simulink model "ORC_test_simu"  (R2018a)
settings: Solver=VariableStepAuto  StartTime=0.0  StopTime=10  RelTol=1e-3
undefined symbols (not defined in the file or in its folder): handle_sink, handle_source, handle_wf, sigbuilder_block
libraries: simulink x1
(part 1 of 3)
settings Model: Creator=njgreen3  LastModifiedBy=njgreen3
settings DebuggingCC: ParameterOverflowMsg=warning

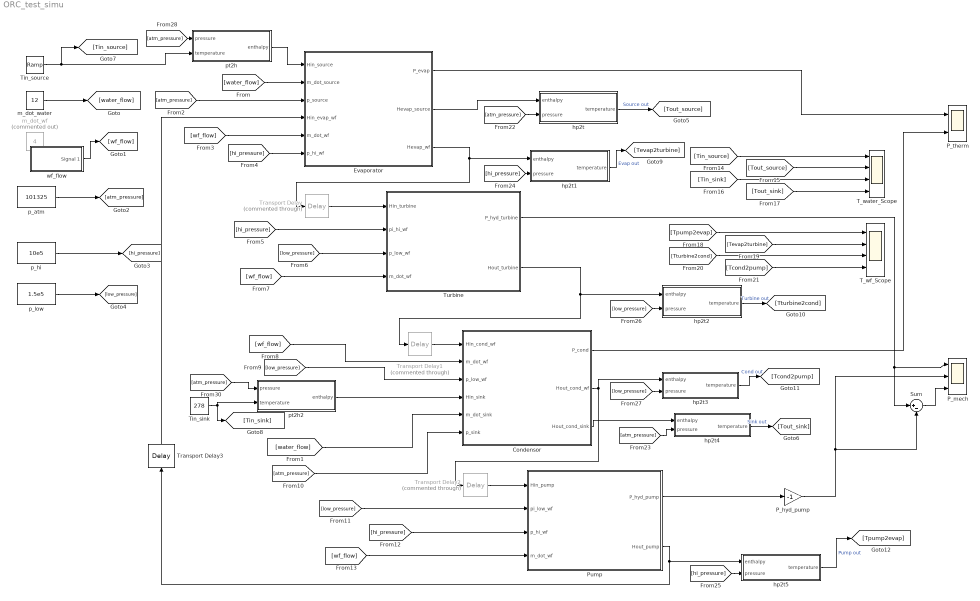
== system ORC_test_simu ==
  Condensor : Subsystem
  Evaporator : Subsystem
  P_hyd_pump : Gain  Gain=-1
  P_mech : Scope  NumInputPorts=3
  P_therm : Scope  NumInputPorts=2
  Pump : Subsystem
  Sum : Sum  Inputs=|+-
  T_water_Scope : Scope  NumInputPorts=4
  T_wf_Scope : Scope  NumInputPorts=4
  Tin_sink : Constant  Value=278
  Tin_source : simulink/Sources/Ramp  slope=0  start=.1  InitialOutput=368
  Transport Delay : TransportDelay  Commented=through  DelayTime=.02  InitialOutput=363
  Transport Delay1 : TransportDelay  Commented=through  DelayTime=.02  InitialOutput=363
  Transport Delay2 : TransportDelay  Commented=through  DelayTime=.02  InitialOutput=306
  Transport Delay3 : TransportDelay  DelayTime=.02  InitialOutput=2.3e+05  TransDelayFeedthrough=on
  Turbine : Subsystem
  hp2t : MATLAB Function  TreatAsAtomicUnit=on  mask{fluid_handle=handle_source}
      mask prompts: fluid_handle "Fluid Handle"
  hp2t1 : MATLAB Function  TreatAsAtomicUnit=on  mask{fluid_handle=handle_wf}
      mask prompts: fluid_handle "Fluid Handle"
  hp2t2 : MATLAB Function  TreatAsAtomicUnit=on  mask{fluid_handle=handle_wf}
      mask prompts: fluid_handle "Fluid Handle"
  hp2t3 : MATLAB Function  TreatAsAtomicUnit=on  mask{fluid_handle=handle_wf}
      mask prompts: fluid_handle "Fluid Handle"
  hp2t4 : MATLAB Function  TreatAsAtomicUnit=on  mask{fluid_handle=handle_sink}
      mask prompts: fluid_handle "Fluid Handle"
  hp2t5 : MATLAB Function  TreatAsAtomicUnit=on  mask{fluid_handle=handle_wf}
      mask prompts: fluid_handle "Fluid Handle"
  m_dot_water : Constant  Value=12
  m_dot_wf : Constant  Commented=on  Value=4
  p_atm : Constant  Value=101325
  p_hi : Constant  Value=10e5
  p_low : Constant  Value=1.5e5
  pt2h : MATLAB Function  TreatAsAtomicUnit=on  mask{fluid_handle=handle_source}
      mask prompts: fluid_handle "Fluid Handle"
  pt2h2 : MATLAB Function  TreatAsAtomicUnit=on  mask{fluid_handle=handle_sink}
      mask prompts: fluid_handle "Fluid Handle"
  wf_flow : Subsystem  Tag=STV Subsys  LoadFcn=sigbuilder_block('load',[319.5 207 550.5 399.75 ]);  StartFcn=sigbuilder_block('start');  StopFcn=sigbuilder_block('stop');  ClipboardFcn=sigbuilder_block('clipboard');  mask(Sigbuilder block){tuvar=[0:10]}
      mask help: Simulink:masks:SigbuilderBlock_MD
      mask init:
      | if ~strcmp(get_param(bdroot(gcbh),'SimulationStatus'),'stopped') tuvar = sigbuilder_block('maskInit'); end
      settings: CopyFcn=sigbuilder_block('copy');  DeleteFcn=sigbuilder_block('delete');  ModelCloseFcn=sigbuilder_block('modelClose');  PreSaveFcn=sigbuilder_block('preSave');  PauseFcn=sigbuilder_block('pause');  ContinueFcn=sigbuilder_block('continue');  NameChangeFcn=sigbuilder_block('namechange');  OpenFcn=sigbuilder_block('open',[437.6 199.2 550.4 400 ]);  CloseFcn=sigbuilder_block('close');
      mask Display: plot(0, 0, 100, 100,[2, 2, 32, 32, 2], [68, 8, 8, 68, 68],[32, 2], [38, 38], [32, 19, 2],[53, 60, 44], [32, 17, 17, 2],[16, 16, 31, 31]);txt = getActiveGroup(gcbh);text(2, 100, txt,'verticalAlignment', 'top');
  wires:
  Evaporator/3(Hevap_wf) -> Transport Delay/1, hp2t1/1(enthalpy)
  Turbine/2(Hout_turbine) -> Transport Delay1/1, hp2t2/1(enthalpy)
  Condensor/2(Hout_cond_wf) -> hp2t3/1(enthalpy), Transport Delay2/1
  Tin_source/1 -> pt2h/2(temperature), [Tin_source]
  m_dot_water/1 -> [water_flow]
  wf_flow/1(Signal 1) -> [wf_flow]
  p_atm/1 -> [atm_pressure]
  p_low/1 -> [low_pressure]
  [water_flow] -> Evaporator/2(m_dot_source)
  [atm_pressure] -> Evaporator/3(p_source)
  [wf_flow] -> Evaporator/5(m_dot_wf)
  [hi_pressure] -> Evaporator/6(p_hi_wf)
  [hi_pressure] -> Turbine/2(pi_hi_wf)
  [low_pressure] -> Turbine/3(p_low_wf)
  [wf_flow] -> Turbine/4(m_dot_wf)
  [wf_flow] -> Condensor/2(m_dot_wf)
  [low_pressure] -> Condensor/3(p_low_wf)
  Tin_sink/1 -> pt2h2/2(temperature), [Tin_sink]
  [water_flow] -> Condensor/5(m_dot_sink)
  [atm_pressure] -> Condensor/6(p_sink)
  [low_pressure] -> Pump/2(pi_low_wf)
  [hi_pressure] -> Pump/3(p_hi_wf)
  [wf_flow] -> Pump/4(m_dot_wf)
  Evaporator/2(Hevap_source) -> hp2t/1(enthalpy)
  Condensor/3(Hout_cond_sink) -> hp2t4/1(enthalpy)
  [Tin_source] -> T_water_Scope/1
  [Tout_source] -> T_water_Scope/2
  [Tin_sink] -> T_water_Scope/3
  [Tout_sink] -> T_water_Scope/4
  [Tpump2evap] -> T_wf_Scope/1
  [Tturbine2cond] -> T_wf_Scope/3
  [Tevap2turbine] -> T_wf_Scope/2
  [Tcond2pump] -> T_wf_Scope/4
  Evaporator/1(P_evap) -> P_therm/1
  Condensor/1(P_cond) -> P_therm/2
  Turbine/1(P_hyd_turbine) -> Sum/1, P_mech/1
  Pump/1(P_hyd_pump) -> P_hyd_pump/1
  Transport Delay/1 -> Turbine/1(Hin_turbine)
  Transport Delay1/1 -> Condensor/1(Hin_cond_wf)
  Transport Delay2/1 -> Pump/1(Hin_pump)
  hp2t/1(temperature) -> [Tout_source]  "Source out"
  hp2t1/1(temperature) -> [Tevap2turbine]  "Evap out"
  hp2t2/1(temperature) -> [Tturbine2cond]  "Turbine out"
  hp2t3/1(temperature) -> [Tcond2pump]  "Cond out"
  hp2t4/1(temperature) -> [Tout_sink]  "Sink out"
  hp2t5/1(temperature) -> [Tpump2evap]  "Pump out"
  [atm_pressure] -> hp2t/2(pressure)
  [atm_pressure] -> hp2t4/2(pressure)
  [hi_pressure] -> hp2t1/2(pressure)
  [hi_pressure] -> hp2t5/2(pressure)
  [low_pressure] -> hp2t2/2(pressure)
  [low_pressure] -> hp2t3/2(pressure)
  pt2h/1(enthalpy) -> Evaporator/1(Hin_source)
  [atm_pressure] -> pt2h/1(pressure)
  Pump/2(Hout_pump) -> Transport Delay3/1, hp2t5/1(enthalpy)
  [atm_pressure] -> pt2h2/1(pressure)
  pt2h2/1(enthalpy) -> Condensor/4(Hin_sink)
  Transport Delay3/1 -> Evaporator/4(Hin_evap_wf)
  P_hyd_pump/1 -> Sum/2, P_mech/2
  p_hi/1 -> [hi_pressure]
  Sum/1 -> P_mech/3

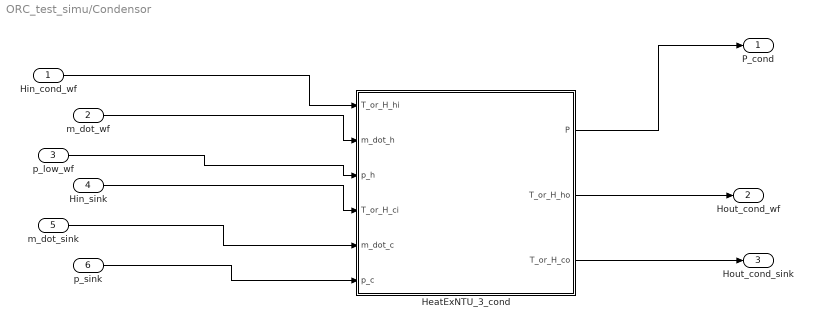
== system ORC_test_simu/Condensor ==
  Hin_cond_wf : Inport
  m_dot_wf : Inport  Port=2
  p_low_wf : Inport  Port=3
  Hin_sink : Inport  Port=4
  m_dot_sink : Inport  Port=5
  p_sink : Inport  Port=6
  HeatExNTU_3_cond : MATLAB Function  Description=|  TreatAsAtomicUnit=on  mask{U=1400, A=18.6, HeatExType=counter, fluid_h=handle_wf, fluid_c=handle_sink, T_or_H=0}
      | %HeatExNTU Summary 
      | %   This function calculates flow and outlet temperatures of a heat exchanger
      | %   using the Number of Transfer Units (NTU) method as described in
      | %   Fundementals of Heat and Mass Transfer by F. P. Incropera, D. P.
      | %   DeWitt, T. L. Bergman & A. S. Lavine. The method can be used when only
      | %   the inlet tempertures are known as opposed to inlet and outlet
      | %   temperatures.
      | %
      | %   This is done by calculating effectiveness which is defined as the ratio
      | %   of actual heat transferred to the maximum possible heat transferred for 
      | %   an infinite length counter-flow heat exchanger with the given inlet
      | %   temperatures. The effectivenes is calculated differently depending on 
      | %   the geometry of exchanger but is always a function of the ratio of heat
      | %   capacity rates as well as the number of transfer units (NTU). The NTU
      | %   depends on the overall heat transfer coefficient, the heat transfer
      | %   area, and the smaller of the two heat capacity rates. 
      | %   
      | %   In the event of a phase change the rate of change of energy required to
      | %   get the fluid just beyond the point of vaporizaion or condensation is
      | %   calculated using the CoolProp function. Then the function is called
      | %   again at the new temperature and the final temperatures and heat rates
      | %   are calucluated using a reduced heat exhange area. I currently assume
      | %   the effected heat transfer area is a half of the original input. This 
      | %   function cannot accurately handle both fluids changing phase because it
      | %   does not check which fluid would change first.
      | % 
      | % Note: The effectiveness is separte from efficiency. The calculations
      | %   assumes an efficiency of 1 where all heat is transferred from the hot
      | %   fluid to the cool fluid or remains within the the fluid. This also
      | %   assumes no fluid is undergoing a change in state, which may not be
      | %   sufficient for my final model.
      | %
      | % This function makes use of the CoolProp wrapper for fluid properties. 
      | % The high level Matlab wrapper cannot handle vector inputs. There ways to
      | % make low level calls interfacing with the DLL so many values can be
      | % determined more quickly, but that is not implented here.
      | % More information about the Matlab wrapper can be found at
      | %   http://www.coolprop.org/coolprop/wrappers/MATLAB/index.html
      | % A list of parameters can be found at 
      | %   http://www.coolprop.org/coolprop/HighLevelAPI.html#parameter-table
      | % A list of fluids can be found at 
      | %   http://www.coolprop.org/fluid_properties/PurePseudoPure.html#list-of-fluids
      | %
      | % Inputs:
      | %   Thi         Hot fluid inlet temperature in Kelvin
      | %   m_dot_h     Hot fluid mass flow rate in kg/s
      | %   p_h         Hot fluid pressure in pa
      | %   fluid_h     Name of Hot fluid (string)
      | %   Tci         Cool fluid inlet temperature in Kelvin
      | %   m_dot_c     Cool fluid mass flow rate in kg/s
      | %   p_c         Cool fluid pressure in pa
      | %   fluid_c     Name of Cool fluid (string)
      | %   HeatExType  String describing the heat exchanger geometry. Currently
      | %               this variable only accepts 'counter' and 'parallel', but
      | %               can be expanded to other exchanger/flow types
      | %               'counter' for counter flow
      | %               'parallel' for parallel
      | %   U           Overall heat transfer coefficient in W/(K m2)
      | %   A           Heat transfer area in m2
      | %
      | % Output:
      | %   P           Rate of heat exchenged (power) in W
      | %   Tho         Hot fluid outlet temperature in input temp units (K)
      | %   Tco         Cool fluid outlet temperature in input tempt units (K)
      mask prompts: U "Heat Transfer Coefficient"; A "Heat Transfer Area"; HeatExType "Heat Exchanger Type"; fluid_h "Hot Fluid Handle"; fluid_c "Cool Fluid Handle"; T_or_H "Temperature(1) or Enthalpy(0)"
  P_cond : Outport
  Hout_cond_wf : Outport  Port=2
  Hout_cond_sink : Outport  Port=3
  wires:
  Hin_cond_wf/1 -> HeatExNTU_3_cond/1(T_or_H_hi)
  m_dot_wf/1 -> HeatExNTU_3_cond/2(m_dot_h)
  p_low_wf/1 -> HeatExNTU_3_cond/3(p_h)
  p_sink/1 -> HeatExNTU_3_cond/6(p_c)
  m_dot_sink/1 -> HeatExNTU_3_cond/5(m_dot_c)
  Hin_sink/1 -> HeatExNTU_3_cond/4(T_or_H_ci)
  HeatExNTU_3_cond/1(P) -> P_cond/1
  HeatExNTU_3_cond/2(T_or_H_ho) -> Hout_cond_wf/1
  HeatExNTU_3_cond/3(T_or_H_co) -> Hout_cond_sink/1

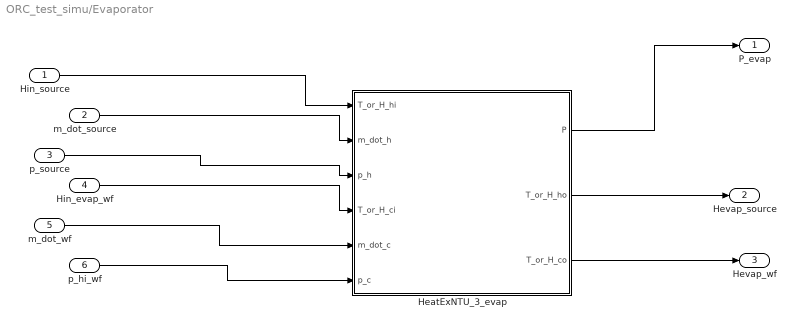
== system ORC_test_simu/Evaporator ==
  Hin_source : Inport
  m_dot_source : Inport  Port=2
  p_source : Inport  Port=3
  Hin_evap_wf : Inport  Port=4
  m_dot_wf : Inport  Port=5
  p_hi_wf : Inport  Port=6
  HeatExNTU_3_evap : MATLAB Function  Description=|  TreatAsAtomicUnit=on  mask{U=1500, A=9.3, HeatExType=counter, fluid_h=handle_source, fluid_c=handle_wf, T_or_H=0}
      | %HeatExNTU Summary 
      | %   This function calculates flow and outlet temperatures of a heat exchanger
      | %   using the Number of Transfer Units (NTU) method as described in
      | %   Fundementals of Heat and Mass Transfer by F. P. Incropera, D. P.
      | %   DeWitt, T. L. Bergman & A. S. Lavine. The method can be used when only
      | %   the inlet tempertures are known as opposed to inlet and outlet
      | %   temperatures.
      | %
      | %   This is done by calculating effectiveness which is defined as the ratio
      | %   of actual heat transferred to the maximum possible heat transferred for 
      | %   an infinite length counter-flow heat exchanger with the given inlet
      | %   temperatures. The effectivenes is calculated differently depending on 
      | %   the geometry of exchanger but is always a function of the ratio of heat
      | %   capacity rates as well as the number of transfer units (NTU). The NTU
      | %   depends on the overall heat transfer coefficient, the heat transfer
      | %   area, and the smaller of the two heat capacity rates. 
      | %   
      | %   In the event of a phase change the rate of change of energy required to
      | %   get the fluid just beyond the point of vaporizaion or condensation is
      | %   calculated using the CoolProp function. Then the function is called
      | %   again at the new temperature and the final temperatures and heat rates
      | %   are calucluated using a reduced heat exhange area. I currently assume
      | %   the effected heat transfer area is a half of the original input. This 
      | %   function cannot accurately handle both fluids changing phase because it
      | %   does not check which fluid would change first.
      | % 
      | % Note: The effectiveness is separte from efficiency. The calculations
      | %   assumes an efficiency of 1 where all heat is transferred from the hot
      | %   fluid to the cool fluid or remains within the the fluid. This also
      | %   assumes no fluid is undergoing a change in state, which may not be
      | %   sufficient for my final model.
      | %
      | % This function makes use of the CoolProp wrapper for fluid properties. 
      | % The high level Matlab wrapper cannot handle vector inputs. There ways to
      | % make low level calls interfacing with the DLL so many values can be
      | % determined more quickly, but that is not implented here.
      | % More information about the Matlab wrapper can be found at
      | %   http://www.coolprop.org/coolprop/wrappers/MATLAB/index.html
      | % A list of parameters can be found at 
      | %   http://www.coolprop.org/coolprop/HighLevelAPI.html#parameter-table
      | % A list of fluids can be found at 
      | %   http://www.coolprop.org/fluid_properties/PurePseudoPure.html#list-of-fluids
      | %
      | % Inputs:
      | %   Thi         Hot fluid inlet temperature in Kelvin
      | %   m_dot_h     Hot fluid mass flow rate in kg/s
      | %   p_h         Hot fluid pressure in pa
      | %   fluid_h     Name of Hot fluid (string)
      | %   Tci         Cool fluid inlet temperature in Kelvin
      | %   m_dot_c     Cool fluid mass flow rate in kg/s
      | %   p_c         Cool fluid pressure in pa
      | %   fluid_c     Name of Cool fluid (string)
      | %   HeatExType  String describing the heat exchanger geometry. Currently
      | %               this variable only accepts 'counter' and 'parallel', but
      | %               can be expanded to other exchanger/flow types
      | %               'counter' for counter flow
      | %               'parallel' for parallel
      | %   U           Overall heat transfer coefficient in W/(K m2)
      | %   A           Heat transfer area in m2
      | %
      | % Output:
      | %   P           Rate of heat exchenged (power) in W
      | %   Tho         Hot fluid outlet temperature in input temp units (K)
      | %   Tco         Cool fluid outlet temperature in input tempt units (K)
      mask prompts: U "Heat Transfer Coefficient"; A "Heat Transfer Area"; HeatExType "Heat Exchanger Type"; fluid_h "Hot Fluid Handle"; fluid_c "Cool Fluid Handle"; T_or_H "Temperature (1) or Enthalpy (0)"
      mask init:
      | % set_param('ORC_test_simu/Evaporator/HeatExNTU_3_block', 'fluid_h', 'Water')
  P_evap : Outport
  Hevap_source : Outport  Port=2
  Hevap_wf : Outport  Port=3
  wires:
  Hin_source/1 -> HeatExNTU_3_evap/1(T_or_H_hi)
  m_dot_source/1 -> HeatExNTU_3_evap/2(m_dot_h)
  p_source/1 -> HeatExNTU_3_evap/3(p_h)
  p_hi_wf/1 -> HeatExNTU_3_evap/6(p_c)
  m_dot_wf/1 -> HeatExNTU_3_evap/5(m_dot_c)
  Hin_evap_wf/1 -> HeatExNTU_3_evap/4(T_or_H_ci)
  HeatExNTU_3_evap/1(P) -> P_evap/1
  HeatExNTU_3_evap/2(T_or_H_ho) -> Hevap_source/1
  HeatExNTU_3_evap/3(T_or_H_co) -> Hevap_wf/1

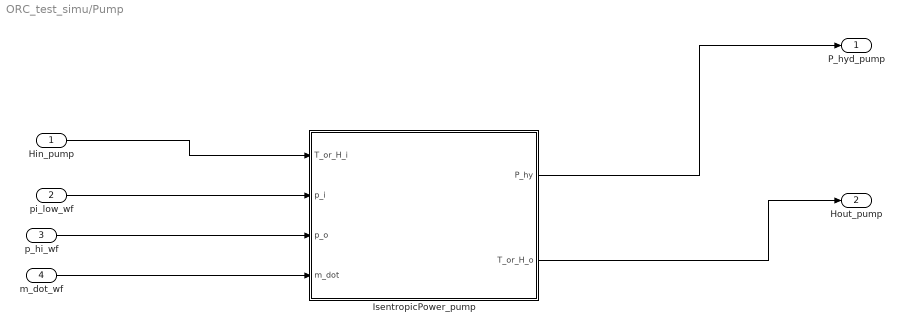
== system ORC_test_simu/Pump ==
  Hin_pump : Inport
  pi_low_wf : Inport  Port=2
  p_hi_wf : Inport  Port=3
  m_dot_wf : Inport  Port=4
  IsentropicPower_pump : MATLAB Function  TreatAsAtomicUnit=on  mask{isen_eff=.78, T_or_H=0, fluid=handle_wf}
      mask prompts: isen_eff "Isentropic Efficiency"; T_or_H "Temperature (1) or Enthalpy (0)"; fluid "Fluid Handle"
  P_hyd_pump : Outport
  Hout_pump : Outport  Port=2
  wires:
  pi_low_wf/1 -> IsentropicPower_pump/2(p_i)
  m_dot_wf/1 -> IsentropicPower_pump/4(m_dot)
  Hin_pump/1 -> IsentropicPower_pump/1(T_or_H_i)
  IsentropicPower_pump/1(P_hy) -> P_hyd_pump/1
  IsentropicPower_pump/2(T_or_H_o) -> Hout_pump/1
  p_hi_wf/1 -> IsentropicPower_pump/3(p_o)

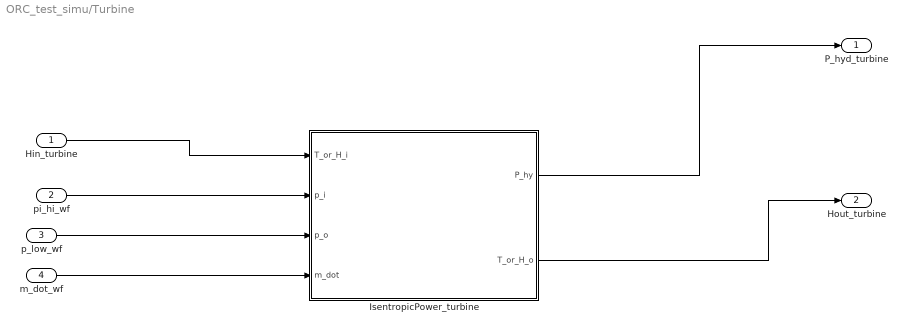
== system ORC_test_simu/Turbine ==
  Hin_turbine : Inport
  pi_hi_wf : Inport  Port=2
  p_low_wf : Inport  Port=3
  m_dot_wf : Inport  Port=4
  IsentropicPower_turbine : MATLAB Function  TreatAsAtomicUnit=on  mask{isen_eff=.78, T_or_H=0, fluid=handle_wf}
      mask prompts: isen_eff "Isentropic Efficiency"; T_or_H "Temperature (1) or Enthalpy (0)"; fluid "Fluid Handle"
  P_hyd_turbine : Outport
  Hout_turbine : Outport  Port=2
  wires:
  pi_hi_wf/1 -> IsentropicPower_turbine/2(p_i)
  m_dot_wf/1 -> IsentropicPower_turbine/4(m_dot)
  Hin_turbine/1 -> IsentropicPower_turbine/1(T_or_H_i)
  IsentropicPower_turbine/1(P_hy) -> P_hyd_turbine/1
  IsentropicPower_turbine/2(T_or_H_o) -> Hout_turbine/1
  p_low_wf/1 -> IsentropicPower_turbine/3(p_o)

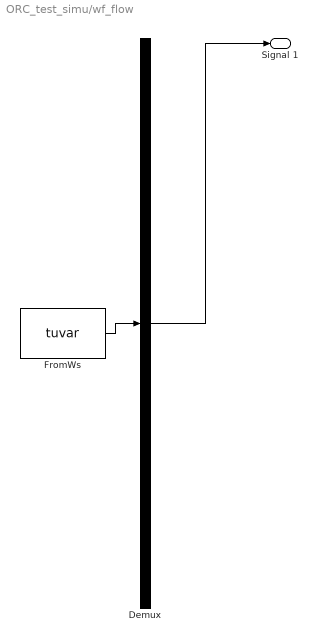
== system ORC_test_simu/wf_flow ==
  Demux : Demux  Tag=STV Demux  Outputs=1
  FromWs : FromWorkspace  Tag=STV FromWs  VariableName=tuvar  SampleTime=0
      SigBuilderData=|
      | common.afterFinalStr = 'Extrapolate'
      | common.sampleTime = 0
      | dataSet.timeRange = [0 10]
      | dataSet.name = 'Group 1'
      | sbobj.Groups.Name = 'Group 1'
      | sbobj.Groups.Signals.Name = 'Signal 1'
      | sbobj.Groups.Signals.XData = [0 1 1 2 2 3 3 4 4 5 5 6 7 8 9 10]
      | sbobj.Groups.Signals.YData = [1.5 1.5 4.9 4.9 9.1 9.1 13.3 13.3 17.2 17.2 20 20 20 20 20 20]
  Signal 1 : Outport  Tag=STV Outport
  wires:
  Demux/1 -> Signal 1/1
  FromWs/1 -> Demux/1

== matlab function ORC_test_simu/Turbine/IsentropicPower_turbine ==
  data: T_or_H_i input; P_hy output; p_i input; p_o input; m_dot input; T_or_H_o output; T_or_H parameter; isen_eff parameter; fluid parameter
function [ P_hy, T_or_H_o ] = IsentropicPower_block( T_or_H_i, p_i, p_o, m_dot, T_or_H,  isen_eff, fluid)
% function [ P_hy ] = IsentropicPower( T_i, T_o, p_i, p_o, m_dot, fluid, isen_eff )
%EXPANDER Summary of this function
%   This process calculates the mechanical power provided or required by a 
%   generic expander device/system. Turbines and other expanders provide
%   mechanical power while pumps and compressors consume it. This is done
%   by calculating the change in enthalpy of fluid and multipying by the 
%   mass flow rate while entropy remains constant.  Non ideal processes are
%   taken into account through the isentropic efficiency.
% 
% Inputs:
%   T_or_H_i    Input temperature in Kelvin or enthalpy in J/kg
%   p_i         Input pressure of the fluid in Pa
%   p_o         Output temperature of the fluid in Pa
%   m_dot       Mass flow rate of the fluid in kg/s 
%   fluid       Initialzed coolprop fluid handle
%   isen_eff    Isentropic efficiency of the device. Expected range: 0-1
%               This input is optional. If it is not provided then it will 
%               be set to 1, which is the efficiency of an ideal isentropic
%               device where entropy is constant.
%               This value is treated differently depending on if there is
%               an increase or decrease in fluid enthalpy. If the enthalpy
%               decreases (energy is extracted from the system) then the
%               efficiency if multiplied by the change in energy because
%               less energy is extracted than the ideal case. If the
%               enthalpy increases (energy in added to the system) then the
%               efficiency is divided by the change in energy because more
%               energy is required than the ideal case.
%   T_or_H      Logical indicating whether the relavent input and output
%               variables are temperature (1) or enthalpy (0)
% 
% Outputs:
%   P_hy        Hydraulic power exctracted or consumed in W. Positive
%               values indicate the system is providing hydraulic power as
%               a turbine or expander. Negative values indicate the system 
%               is consuming hydraulic power as a compressor or pump.
%   T_or_H_o    Output temperature in Kelvin or enthalpy in J/kg

% This function makes use of the CoolProp wrapper for fluid properties. 
% The high level Matlab wrapper cannot handle vector inputs. There ways to
% make low level calls interfacing with the DLL so many values can be
% determined more quickly, but that is not implented here.
% More information about the Matlab wrapper can be found at
%   http://www.coolprop.org/coolprop/wrappers/MATLAB/index.html
% A list of parameters can be found at 
%   http://www.coolprop.org/coolprop/HighLevelAPI.html#parameter-table
% A list of fluids can be found at 
%   http://www.coolprop.org/fluid_properties/PurePseudoPure.html#list-of-fluids

% initailize certain parameters used to call coolprop library
buffer_size = 255;
ierr = 0;
b = (1:1:buffer_size);
herr= char(b);
coder.extrinsic('calllib') 
coder.extrinsic('libpointer') 

% All the input signals should be the same size, so it shouldn't matter
% which one is used to obtain signal length
var_length = length(T_or_H_i);
% T_or_H_i

% fluid_h = 'water';
% fluid = 'R245fa';
% % initialize handles for hot and cool fluids
% [fluid, ~] = calllib('coolprop','AbstractState_factory',backend,fluid,ierr,herr,buffer_size);

% determine input parameter pair indecies for coolprop calls
% [pq_ind,~] = calllib('coolprop','get_input_pair_index','PQ_INPUTS'); %pressure and Mass vapor quality
[pt_ind,~] = calllib('coolprop','get_input_pair_index','PT_INPUTS'); %pressure and temperature
[hp_ind,~] = calllib('coolprop','get_input_pair_index','HmassP_INPUTS'); %Mass specific enthalpy and pressure
[ps_ind,~] = calllib('coolprop','get_input_pair_index','PSmass_INPUTS'); %pressure and Mass specific entropy

% determine output parameter indecies for coolprop calls
[t_ind, ~] = calllib('coolprop','get_param_index','T'); %temperature
[s_ind, ~] = calllib('coolprop','get_param_index','S'); %Mass specific entropy
[h_ind, ~] = calllib('coolprop','get_param_index','Hmass'); %Mass specific enthalpy
% [c_ind, ~] = calllib('coolprop','get_param_index','Cpmass'); %Mass specific constant pressure specific heat

% find pointer location of pressure input and output values
p_i_Ptr = libpointer('doublePtr',p_i);
p_o_Ptr = libpointer('doublePtr',p_o);

% % Check inputs
% if nargin < 7
% %   Set equal to 1 if isen_eff is not in input
%     isen_eff = 1;
%     
%     if nargin < 6
%         error(message('NotEnoughInputs'));
%     end
% end
% % check if isen_eff is in range
% if isen_eff > 1 || isen_eff < 0
%     error(message('isen_eff is out of range'));
% end

% T_or_H = 'T';
% Ensure temperature/enthalpy input variables are delt with appropriately
% if upper(T_or_H) == 'T' %|| 'TEMPERATURE'
if T_or_H %== 'T' %|| 'TEMPERATURE'
% Assume given temperature values are not at vaporization/condensation.
% Initialize T and H inputs
    T_i = T_or_H_i;
    T_i_Ptr = libpointer('doublePtr',T_i);
    H_i = zeros(var_length,1); % initialized to 0 temporarily
    H_i_Ptr = libpointer('doublePtr',H_i);
% Update values located at Hhi and Hci pointer locations
    calllib('coolprop','AbstractState_update_and_1_out', fluid, pt_ind, p_i_Ptr, T_i_Ptr, var_length, h_ind, H_i_Ptr, ierr,herr,buffer_size);
% Set Hhi & Hci to values stored at pointer location
    H_i = get(H_i_Ptr,'Value');
    
else%if T_or_H == 'H' %|| 'ENTHALPY'
% Enthalpy values can be in vaporization/condensation region  
% Initialize H values
    H_i = T_or_H_i;
    H_i_Ptr = libpointer('doublePtr',H_i);
% else
%     error('Please specify whether input uses variables of Temperature or Enthalpy.')
end

% Input entropy in J/kg/K
% Initialize pointer locations for relevant variables
S_i_Ptr = libpointer('doublePtr', zeros(var_length,1)); 
% Update values at S_i pointer location
calllib('coolprop','AbstractState_update_and_1_out', fluid, hp_ind, H_i_Ptr, p_i_Ptr, var_length, s_ind, S_i_Ptr, ierr,herr,buffer_size);
% Set S_i to values stored at pointer location
% S_i = get(S_i_Ptr,'Value');

% Ideal Output entropy is equal to input entropy 
% Ideal Output enthalpy in J/kg and temperature
H_o_ideal = zeros(var_length,1);
H_o_ideal_Ptr = libpointer('doublePtr',H_o_ideal);
% Update values located at Hhi and Hci pointer locations
calllib('coolprop','AbstractState_update_and_1_out', fluid, ps_ind, p_o_Ptr, S_i_Ptr, var_length, h_ind, H_o_ideal_Ptr, ierr,herr,buffer_size);
% Set H_o_ideal to values stored at pointer location
H_o_ideal = get(H_o_ideal_Ptr,'Value');
% T_o_ideal = CoolProp.PropsSI('T', 'P', p_o, 'S', S_i, fluid);

% Calculate Ideal power consumed/provided
P_ideal = m_dot.*(H_i - H_o_ideal);

% Initialize hydrolic power variable
P_hy = zeros(var_length,1);
%   If positive then the system is providing power as a turbine
%   or expander.
%   This means the actual power provided is less than the ideal power
P_hy(P_ideal > 0) = isen_eff.*P_ideal(P_ideal > 0);

%   If negative then the system is consuming power as a
%   compressor or pump.
%   This means the actual power consumed is greater than the ideal power.
P_hy(P_ideal < 0) = P_ideal(P_ideal < 0)./isen_eff;

% %   If the ideal power consumed/provided is 0 then either the fluid did not 
% %   undergo any change or some (non-ideal) work was consumed to change it's
% %   state
%     warning('Actual mechanical power cannot be determined from the information provided.');
%     P_hy = NaN;
%     T_o = T_i;
%     return;


H_o = H_i - P_hy./m_dot;
H_o_Ptr = libpointer('doublePtr',H_o);
% T_o = CoolProp.PropsSI('T', 'P', p_o, 'H', H_o, fluid);

% Ensure temperature/enthalpy input variables are delt with appropriately
% if upper(T_or_H) == 'T' %|| 'TEMPERATURE'
if T_or_H %== 'T' %|| 'TEMPERATURE'
% Assume given temperature values are not at vaporization/condensation
    T_or_H_o = zeros(var_length,1);
    T_or_H_o_Ptr = libpointer('doublePtr',T_or_H_o);
    calllib('coolprop','AbstractState_update_and_1_out', fluid, hp_ind, H_o_Ptr, p_o_Ptr, var_length, t_ind, T_or_H_o_Ptr, ierr,herr,buffer_size);
    T_or_H_o = get(T_or_H_o_Ptr,'Value');
    
else%if upper(T_or_H) == 'H' %|| 'ENTHALPY'
% Enthalpy values can be in vaporization/condensation region    
    T_or_H_o = H_o;
end
% calllib('coolprop','AbstractState_free', fluid, ierr,herr,buffer_size);
end
